simulink model "System2016"  (R2016b)
settings: Solver=ode45  StartTime=0.0  StopTime=3  RelTol=1e-3  EnableMultiTasking=on
libraries: powerlib x4, simulink x2, powerlib_meascontrol x1
settings Model: Creator=Administrator  LastModifiedBy=Administrator
settings DataIOCC: LimitDataPoints=on  SaveFormat=Array
settings OptimizationCC: LifeSpan=inf
settings DebuggingCC: SolverPrmCheckMsg=warning  SFUnexpectedBacktrackingDiag=warning  SFNoUnconditionalDefaultTransitionDiag=warning  SFExecutionAtInitializationDiag=none
settings HardwareCC: ProdBitPerPointer=32  ProdBitPerSizeT=32  ProdBitPerPtrDiffT=32  ProdLargestAtomicFloat=None  ProdIntDivRoundTo=Undefined  ProdEndianess=Unspecified  ProdWordSize=32  ProdHWDeviceType=32-bit Generic
settings ModelReferenceCC: PropagateSignalLabelsOutOfModel=off
settings GRTTargetCC: TargetLangStandard=C89/C90 (ANSI)  GeneratePreprocessorConditionals=Disable all
settings ConfigComp: CovMetricSettings=dw  CovHtmlReporting=on  CovSaveCumulativeToWorkspaceVar=on  CovSaveSingleToWorkspaceVar=on  CovExternalEMLEnable=off  CovSFcnEnable=off

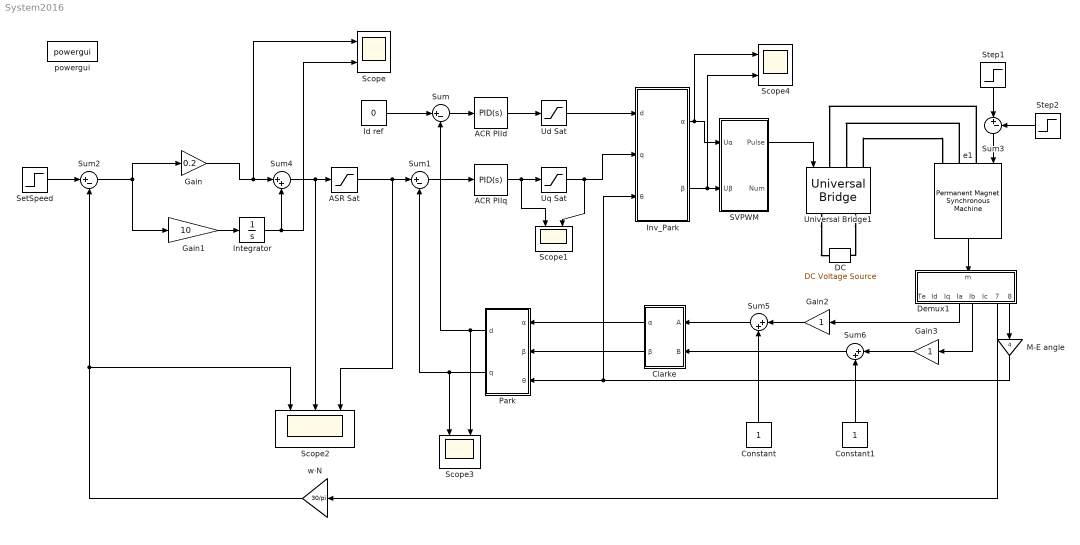
== system System2016 ==
  " e1" : powerlib/Machines/Permanent Magnet Synchronous Machine  NbPhases=3  FluxDistribution=Sinusoidal  RotorType=Round  MechanicalLoad=Torque Tm  PresetModel=No  ShowDetailedParameters=on  MeasurementBus=off  Resistance=1  Inductance=8.5e-3  dqInductances=[8.5e-3,8.5e-3]  La=0.01  MachineConstant=Flux linkage established by magnets (V.s)  Flux=0.1827  VoltageCst=132.5525  TorqueCst=1.0962  Flat=120  Mechanical=[0.006 0.0003035 4 0]  PolePairs=4  InitialConditions=[0,0, 0,0]  InitialConditions5ph=[0 0 0 0 0 0]  TsPowergui=0  TsBlock=-1  RefAngle=Aligned with phase A axis (original Park)
  ACR PIId : simulink/Continuous/PID Controller  Controller=PID  TimeDomain=Continuous-time  SampleTime=-1  IntegratorMethod=Forward Euler  FilterMethod=Forward Euler  Form=Parallel  UseFilter=on  ControllerParametersSource=internal  P=45  I=23  D=0  N=100  InitialConditionSource=internal  InitialConditionForIntegrator=0  InitialConditionForFilter=0  ExternalReset=none  LimitOutput=off  UpperSaturationLimit=inf  LowerSaturationLimit=-inf  LinearizeAsGain=on  AntiWindupMode=none  Kb=1  TrackingMode=off  Kt=1  PParamMin=[]  PParamMax=[]  IParamMin=[]  IParamMax=[]  DParamMin=[]  DParamMax=[]  NParamMin=[]  NParamMax=[]  KbParamMin=[]  KbParamMax=[]  KtParamMin=[]  KtParamMax=[]  POutMin=[]  POutMax=[]  IOutMin=[]  IOutMax=[]  DOutMin=[]  DOutMax=[]  NOutMin=[]  NOutMax=[]  KbOutMin=[]  KbOutMax=[]  KtOutMin=[]  KtOutMax=[]  IntegratorOutMin=[]  IntegratorOutMax=[]  FilterOutMin=[]  FilterOutMax=[]  SumOutMin=[]  SumOutMax=[]  SumI1OutMin=[]  SumI1OutMax=[]  SumI2OutMin=[]  SumI2OutMax=[]  SumI3OutMin=[]  SumI3OutMax=[]  SumDOutMin=[]  SumDOutMax=[]  SaturationOutMin=[]  SaturationOutMax=[]  IntegratorContinuousStateAttributes=''  IntegratorStateMustResolveToSignalObject=off  IntegratorRTWStateStorageClass=Auto  FilterContinuousStateAttributes=''  FilterStateMustResolveToSignalObject=off  FilterRTWStateStorageClass=Auto  DifferentiatorICPrevScaledInput=0  DifferentiatorOutMin=[]  DifferentiatorOutMax=[]
  ACR PIIq : simulink/Continuous/PID Controller  Controller=PID  TimeDomain=Continuous-time  SampleTime=-1  IntegratorMethod=Forward Euler  FilterMethod=Forward Euler  Form=Parallel  UseFilter=on  ControllerParametersSource=internal  P=32  I=23  D=0  N=100  InitialConditionSource=internal  InitialConditionForIntegrator=0  InitialConditionForFilter=0  ExternalReset=none  LimitOutput=off  UpperSaturationLimit=inf  LowerSaturationLimit=-inf  LinearizeAsGain=on  AntiWindupMode=none  Kb=1  TrackingMode=off  Kt=1  PParamMin=[]  PParamMax=[]  IParamMin=[]  IParamMax=[]  DParamMin=[]  DParamMax=[]  NParamMin=[]  NParamMax=[]  KbParamMin=[]  KbParamMax=[]  KtParamMin=[]  KtParamMax=[]  POutMin=[]  POutMax=[]  IOutMin=[]  IOutMax=[]  DOutMin=[]  DOutMax=[]  NOutMin=[]  NOutMax=[]  KbOutMin=[]  KbOutMax=[]  KtOutMin=[]  KtOutMax=[]  IntegratorOutMin=[]  IntegratorOutMax=[]  FilterOutMin=[]  FilterOutMax=[]  SumOutMin=[]  SumOutMax=[]  SumI1OutMin=[]  SumI1OutMax=[]  SumI2OutMin=[]  SumI2OutMax=[]  SumI3OutMin=[]  SumI3OutMax=[]  SumDOutMin=[]  SumDOutMax=[]  SaturationOutMin=[]  SaturationOutMax=[]  IntegratorContinuousStateAttributes=''  IntegratorStateMustResolveToSignalObject=off  IntegratorRTWStateStorageClass=Auto  FilterContinuousStateAttributes=''  FilterStateMustResolveToSignalObject=off  FilterRTWStateStorageClass=Auto  DifferentiatorICPrevScaledInput=0  DifferentiatorOutMin=[]  DifferentiatorOutMax=[]
  ASR Sat : Saturate  UpperLimit=2  LowerLimit=-2
  Clarke : Subsystem
  Constant : Constant
  Constant1 : Constant
  DC : powerlib/Electrical Sources/DC Voltage Source  Amplitude=50  Measurements=None
  Demux1 : Subsystem
  Gain : Gain  Gain=0.2
  Gain1 : Gain  Gain=10
  Gain2 : Gain
  Gain3 : Gain
  Id ref : Constant  Value=0
  Integrator : Integrator
  Inv_Park : Subsystem
  M-E angle : Gain  Gain=4
  Park : Subsystem
  "SVPWM " : Subsystem
  Scope{,1,3..4} (4 alike) : Scope  NumInputPorts=2
  Scope2 : Scope  NumInputPorts=3
  SetSpeed : Step  Time=0  Before=40  After=40  SampleTime=0
  Step1 : Step  Before=1  After=1.5  SampleTime=0
  Step2 : Step  Time=1.05  After=0.5  SampleTime=0
  Sum{,1..3} (4 alike) : Sum  Inputs=|+-
  Sum4 : Sum  Inputs=|++
  Sum5 : Sum  Inputs=|++
  Sum6 : Sum  Inputs=|++
  Ud Sat : Saturate  UpperLimit=38  LowerLimit=-38
  Universal Bridge1 : powerlib/Power Electronics/Universal Bridge  Arms=3  SnubberResistance=1e5  SnubberCapacitance=inf  Device=IGBT / Diodes  Ron=1e-3  Lon=0  ForwardVoltages="[  0  0  ]"  ForwardVoltage=0  GTOparameters=[ 10e-6 , 20e-6 ]  IGBTparameters=[ 1e-6 , 2e-6 ]  Measurements=None  Measurements_2=None  converterType=Rectifier
  Uq Sat : Saturate  UpperLimit=38  LowerLimit=-38
  powergui : powerlib/powergui  SimulationMode=Continuous  SolverType=Tustin  SampleTime=50e-6  frequency=60  SPID=off  DisableSnubberDevices=off  DisableRonSwitches=off  DisableVfSwitches=off  SwTol=0  DisplayEquations=off  Interpol=off  ExternalGateDelay=off  methode=off  Ts=0  FunctionMessages=off  echomessages=off  HookPort=off  EnableUseOfTLC=off  x0status=blocks  frequencyindice=0  Pbase=100e6  ErrMax=1e-4  Iterations=50  UnitsV=kV  UnitsW=MW  buscounter=0  RestoreLinks=warning  ResistiveCurrentMeasurement=off  Frange=[0:2:500]  Ylog=off  Xlog=on  ShowGrid=off  save=off  variable=ZData  structure=0  ZoomFFT=on  StartTime=0.0  cycles=1  DisplayStyle=1  fundamental=60  FreqAxis=off  MaxFrequency=1000  frequencyindicesteady=1  RmsSteady=1  display=off
  w·N : Gain  Gain=30/pi
  wires:
  "SVPWM "/1(Pulse) -> Universal Bridge1/1
  Inv_Park/1(α) -> Scope4/1, "SVPWM "/1(Uα)
  Inv_Park/2(β) -> Scope4/2, "SVPWM "/2(Uβ)
  Sum/1 -> ACR PIId/1
  Sum1/1 -> ACR PIIq/1
  Id ref/1 -> Sum/1
  SetSpeed/1 -> Sum2/1
  Demux1/8(thetam) -> M-E angle/1
  Demux1/7(wm) -> w·N/1
  " e1"/1 -> Demux1/1(m)
  M-E angle/1 -> Park/3(θ), Inv_Park/3(θ)
  Clarke/1(α) -> Park/1(α)
  Clarke/2(β) -> Park/2(β)
  w·N/1 -> Sum2/2, Scope2/1
  Ud Sat/1 -> Inv_Park/1(d)
  Uq Sat/1 -> Scope1/2, Inv_Park/2(q)
  ACR PIIq/1 -> Scope1/1, Uq Sat/1
  ACR PIId/1 -> Ud Sat/1
  Park/1(d) -> Scope3/2, Sum/2
  Park/2(q) -> Scope3/1, Sum1/2
  ASR Sat/1 -> Scope2/3, Sum1/1
  Step1/1 -> Sum3/1
  Sum3/1 -> " e1"/1
  Step2/1 -> Sum3/2
  Sum4/1 -> Scope2/2, ASR Sat/1
  Integrator/1 -> Scope/2, Sum4/2
  Gain1/1 -> Integrator/1
  Sum2/1 -> Gain/1, Gain1/1
  Gain/1 -> Scope/1, Sum4/1
  Sum5/1 -> Clarke/1(A)
  Sum6/1 -> Clarke/2(B)
  Demux1/5(Ib) -> Gain3/1
  Demux1/4(Ia) -> Gain2/1
  Gain2/1 -> Sum5/1
  Gain3/1 -> Sum6/1
  Constant/1 -> Sum5/2
  Constant1/1 -> Sum6/2
  connections:
  " e1"/LConn1 -- Universal Bridge1/LConn1
  " e1"/LConn2 -- Universal Bridge1/LConn2
  Universal Bridge1/LConn3 -- " e1"/LConn3
  Universal Bridge1/RConn1 -- DC/RConn1
  Universal Bridge1/RConn2 -- DC/LConn1

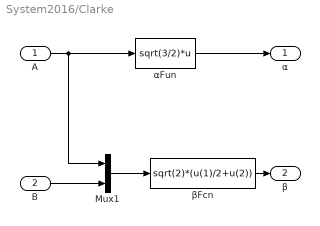
== system System2016/Clarke ==
  A : Inport
  B : Inport  Port=2
  Mux1 : Mux  Inputs=2
  αFun : Fcn  Expr=sqrt(3/2)*u
  βFcn : Fcn  Expr=sqrt(2)*(u(1)/2+u(2))
  α : Outport
  β : Outport  Port=2
  wires:
  A/1 -> Mux1/1, αFun/1
  αFun/1 -> α/1
  B/1 -> Mux1/2
  Mux1/1 -> βFcn/1
  βFcn/1 -> β/1

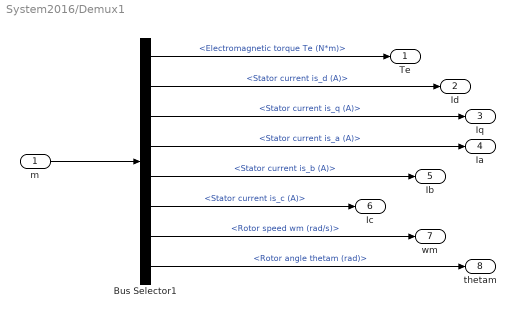
== system System2016/Demux1 ==
  m : Inport
  Bus Selector1 : BusSelector  OutputSignals=Electromagnetic torque Te (N*m),Stator current is_d (A),Stator current is_q (A),Stator current is_a (A),Stator current is_b (A),Stator current is_c (A),Rotor speed wm (rad/s),Rotor angle thetam (rad)
  Te : Outport
  Id : Outport  Port=2
  Iq : Outport  Port=3
  Ia : Outport  Port=4
  Ib : Outport  Port=5
  Ic : Outport  Port=6
  wm : Outport  Port=7
  thetam : Outport  Port=8
  wires:
  m/1 -> Bus Selector1/1
  Bus Selector1/4 -> Ia/1  "<Stator current is_a (A)>"
  Bus Selector1/5 -> Ib/1  "<Stator current is_b (A)>"
  Bus Selector1/6 -> Ic/1  "<Stator current is_c (A)>"
  Bus Selector1/7 -> wm/1  "<Rotor speed wm (rad/s)>"
  Bus Selector1/8 -> thetam/1  "<Rotor angle thetam (rad)>"
  Bus Selector1/1 -> Te/1  "<Electromagnetic torque Te (N*m)>"
  Bus Selector1/2 -> Id/1  "<Stator current is_d (A)>"
  Bus Selector1/3 -> Iq/1  "<Stator current is_q (A)>"

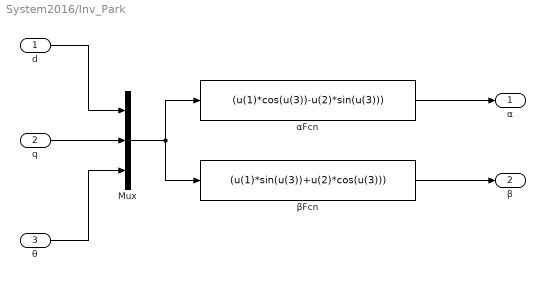
== system System2016/Inv_Park ==
  d : Inport
  q : Inport  Port=2
  θ : Inport  Port=3
  Mux : Mux  Inputs=3
  αFcn : Fcn  Expr=(u(1)*cos(u(3))-u(2)*sin(u(3)))
  βFcn : Fcn  Expr=(u(1)*sin(u(3))+u(2)*cos(u(3)))
  α : Outport
  β : Outport  Port=2
  wires:
  d/1 -> Mux/1
  q/1 -> Mux/2
  θ/1 -> Mux/3
  αFcn/1 -> α/1
  βFcn/1 -> β/1
  Mux/1 -> βFcn/1, αFcn/1

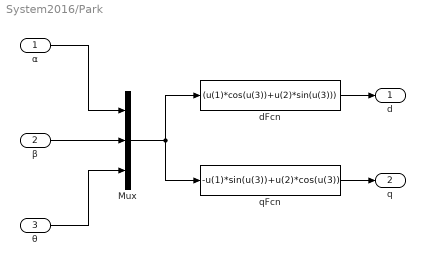
== system System2016/Park ==
  α : Inport
  β : Inport  Port=2
  θ : Inport  Port=3
  Mux : Mux  Inputs=3
  dFcn : Fcn  Expr=(u(1)*cos(u(3))+u(2)*sin(u(3)))
  qFcn : Fcn  Expr=-u(1)*sin(u(3))+u(2)*cos(u(3))
  d : Outport
  q : Outport  Port=2
  wires:
  α/1 -> Mux/1
  β/1 -> Mux/2
  θ/1 -> Mux/3
  dFcn/1 -> d/1
  qFcn/1 -> q/1
  Mux/1 -> qFcn/1, dFcn/1

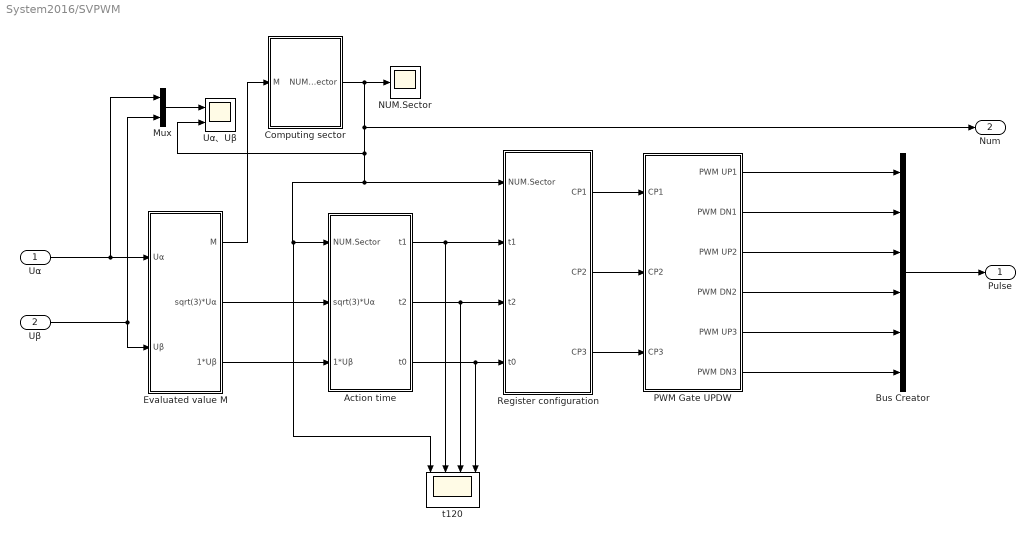
== system System2016/SVPWM  ==
  Uα : Inport
  Uβ : Inport  Port=2
  Action time : Subsystem
  Bus Creator : BusCreator  Inputs=6
  Computing sector : Subsystem
  Evaluated value M : Subsystem
  Mux : Mux  Inputs=2
  NUM.Sector : Scope
  PWM Gate UPDW : Subsystem
  Register configuration : Subsystem
  Uα、Uβ : Scope  NumInputPorts=2
  t120 : Scope  NumInputPorts=4
  Pulse : Outport
  Num : Outport  Port=2
  wires:
  Evaluated value M/1(M) -> Computing sector/1(M)
  Computing sector/1(NUM.Sector) -> NUM.Sector/1, Num/1, Uα、Uβ/2, t120/1, Action time/1(NUM.Sector), Register configuration/1(NUM.Sector)
  Evaluated value M/2(sqrt(3)*Uα) -> Action time/2(sqrt(3)*Uα)
  Evaluated value M/3(1*Uβ) -> Action time/3(1*Uβ)
  Action time/1(t1) -> t120/2, Register configuration/2(t1)
  Action time/2(t2) -> t120/3, Register configuration/3(t2)
  Action time/3(t0) -> t120/4, Register configuration/4(t0)
  Register configuration/1(CP1) -> PWM Gate UPDW/1(CP1)
  Register configuration/2(CP2) -> PWM Gate UPDW/2(CP2)
  Register configuration/3(CP3) -> PWM Gate UPDW/3(CP3)
  PWM Gate UPDW/1(PWM UP1) -> Bus Creator/1
  Uα/1 -> Mux/1, Evaluated value M/1(Uα)
  Uβ/1 -> Mux/2, Evaluated value M/2(Uβ)
  Mux/1 -> Uα、Uβ/1
  Bus Creator/1 -> Pulse/1
  PWM Gate UPDW/2(PWM DN1) -> Bus Creator/2
  PWM Gate UPDW/3(PWM UP2) -> Bus Creator/3
  PWM Gate UPDW/4(PWM DN2) -> Bus Creator/4
  PWM Gate UPDW/5(PWM UP3) -> Bus Creator/5
  PWM Gate UPDW/6(PWM DN3) -> Bus Creator/6

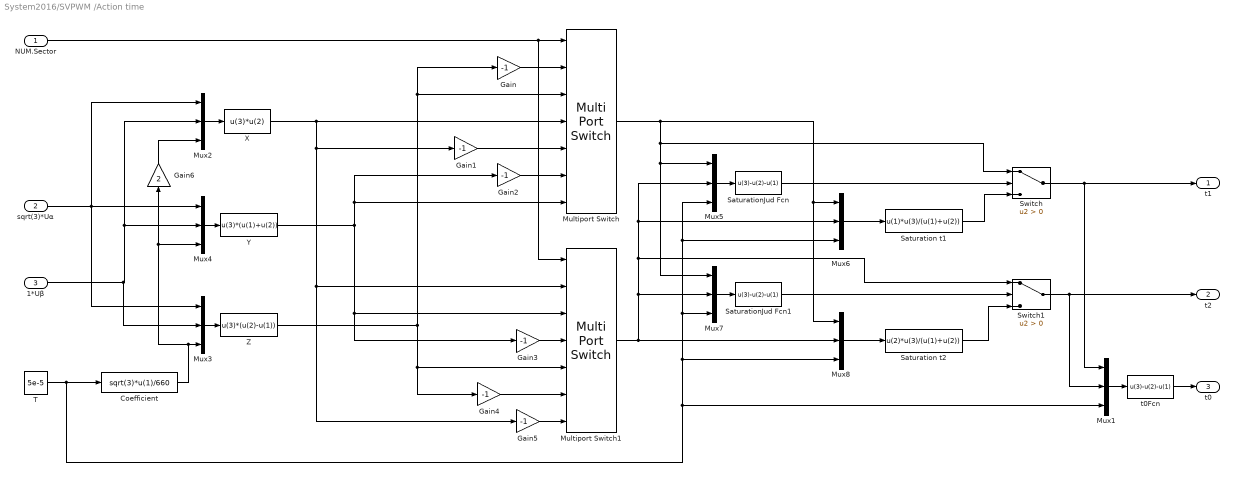
== system System2016/SVPWM /Action time ==
  NUM.Sector : Inport
  sqrt(3)*Uα : Inport  Port=2
  1*Uβ : Inport  Port=3
  Coefficient : Fcn  Expr=sqrt(3)*u(1)/660
  Gain{,1..5} (6 alike) : Gain  Gain=-1
  Gain6 : Gain  Gain=2
  Multiport Switch : MultiPortSwitch  Inputs=6
  Multiport Switch1 : MultiPortSwitch  Inputs=6
  Mux{1..8} (8 alike) : Mux  Inputs=3
  Saturation t1 : Fcn  Expr=u(1)*u(3)/(u(1)+u(2))
  Saturation t2 : Fcn  Expr=u(2)*u(3)/(u(1)+u(2))
  SaturationJud Fcn : Fcn  Expr=u(3)-u(2)-u(1)
  SaturationJud Fcn1 : Fcn  Expr=u(3)-u(2)-u(1)
  Switch : Switch  Criteria=u2 > Threshold
  Switch1 : Switch  Criteria=u2 > Threshold
  T : Constant  Value=5e-5
  X : Fcn  Expr=u(3)*u(2)
  Y : Fcn  Expr=u(3)*(u(1)+u(2))
  Z : Fcn  Expr=u(3)*(u(2)-u(1))
  t0Fcn : Fcn  Expr=u(3)-u(2)-u(1)
  t1 : Outport
  t2 : Outport  Port=2
  t0 : Outport  Port=3
  wires:
  NUM.Sector/1 -> Multiport Switch1/1, Multiport Switch/1
  T/1 -> Coefficient/1, Mux1/3, Mux8/3, Mux7/3, Mux5/3, Mux6/3
  Mux1/1 -> t0Fcn/1
  t0Fcn/1 -> t0/1
  sqrt(3)*Uα/1 -> Mux3/1, Mux4/1, Mux2/1
  1*Uβ/1 -> Mux3/2, Mux4/2, Mux2/2
  Coefficient/1 -> Mux4/3, Gain6/1, Mux3/3
  Mux2/1 -> X/1
  Mux4/1 -> Y/1
  Mux3/1 -> Z/1
  Gain/1 -> Multiport Switch/2
  Gain1/1 -> Multiport Switch/5
  Gain2/1 -> Multiport Switch/6
  Gain3/1 -> Multiport Switch1/4
  Gain4/1 -> Multiport Switch1/6
  Gain5/1 -> Multiport Switch1/7
  Z/1 -> Gain/1, Multiport Switch/3, Multiport Switch1/5, Gain4/1
  X/1 -> Gain1/1, Multiport Switch1/2, Gain5/1, Multiport Switch/4
  Y/1 -> Multiport Switch/7, Gain2/1, Gain3/1, Multiport Switch1/3
  Multiport Switch/1 -> Mux8/1, Mux6/1, Switch/1, Mux7/1, Mux5/1
  Multiport Switch1/1 -> Mux7/2, Switch1/1, Mux6/2, Mux5/2, Mux8/2
  Mux5/1 -> SaturationJud Fcn/1
  SaturationJud Fcn/1 -> Switch/2
  Switch/1 -> Mux1/1, t1/1
  Saturation t1/1 -> Switch/3
  Mux6/1 -> Saturation t1/1
  Mux7/1 -> SaturationJud Fcn1/1
  Switch1/1 -> Mux1/2, t2/1
  Mux8/1 -> Saturation t2/1
  SaturationJud Fcn1/1 -> Switch1/2
  Saturation t2/1 -> Switch1/3
  Gain6/1 -> Mux2/3

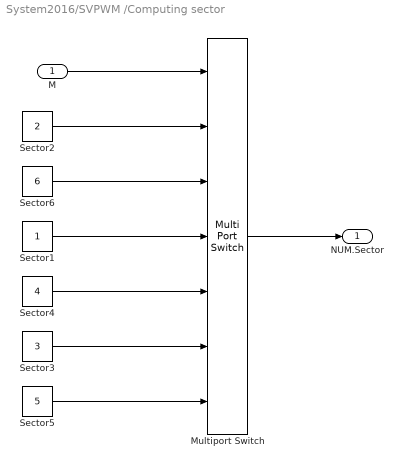
== system System2016/SVPWM /Computing sector ==
  M : Inport
  Multiport Switch : MultiPortSwitch  Inputs=6
  Sector1 : Constant
  Sector2 : Constant  Value=2
  Sector3 : Constant  Value=3
  Sector4 : Constant  Value=4
  Sector5 : Constant  Value=5
  Sector6 : Constant  Value=6
  NUM.Sector : Outport
  wires:
  M/1 -> Multiport Switch/1
  Sector2/1 -> Multiport Switch/2
  Sector6/1 -> Multiport Switch/3
  Sector1/1 -> Multiport Switch/4
  Sector4/1 -> Multiport Switch/5
  Sector3/1 -> Multiport Switch/6
  Sector5/1 -> Multiport Switch/7
  Multiport Switch/1 -> NUM.Sector/1

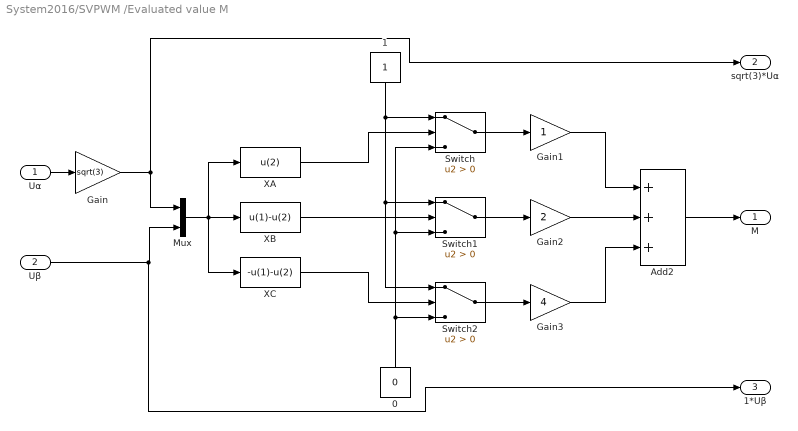
== system System2016/SVPWM /Evaluated value M ==
  Uα : Inport
  Uβ : Inport  Port=2
  0 : Constant  Value=0
  1 : Constant
  Add2 : Sum  Inputs=+++
  Gain : Gain  Gain=sqrt(3)
  Gain1 : Gain
  Gain2 : Gain  Gain=2
  Gain3 : Gain  Gain=4
  Mux : Mux  Inputs=2
  Switch : Switch  Criteria=u2 > Threshold
  Switch1 : Switch  Criteria=u2 > Threshold
  Switch2 : Switch  Criteria=u2 > Threshold
  XA : Fcn  Expr=u(2)
  XB : Fcn  Expr=u(1)-u(2)
  XC : Fcn  Expr=-u(1)-u(2)
  M : Outport
  sqrt(3)*Uα : Outport  Port=2
  1*Uβ : Outport  Port=3
  wires:
  Uβ/1 -> 1*Uβ/1, Mux/2
  Mux/1 -> XA/1, XB/1, XC/1
  XB/1 -> Switch1/2
  XA/1 -> Switch/2
  XC/1 -> Switch2/2
  0/1 -> Switch2/3, Switch1/3, Switch/3
  1/1 -> Switch/1, Switch1/1, Switch2/1
  Switch/1 -> Gain1/1
  Switch1/1 -> Gain2/1
  Switch2/1 -> Gain3/1
  Gain1/1 -> Add2/1
  Gain2/1 -> Add2/2
  Gain3/1 -> Add2/3
  Add2/1 -> M/1
  Uα/1 -> Gain/1
  Gain/1 -> Mux/1, sqrt(3)*Uα/1

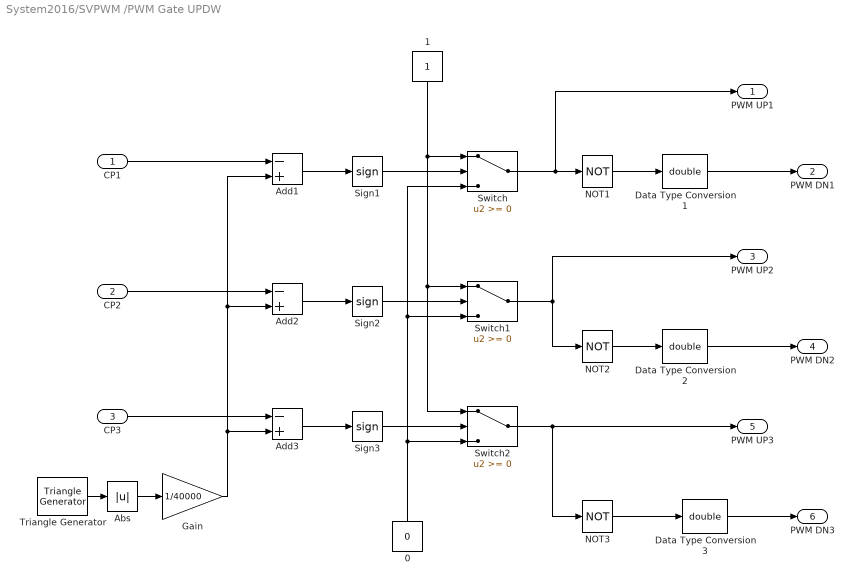
== system System2016/SVPWM /PWM Gate UPDW ==
  CP1 : Inport
  CP2 : Inport  Port=2
  CP3 : Inport  Port=3
  0 : Constant  Value=0
  1 : Constant
  Abs : Abs
  Add1 : Sum  Inputs=-+
  Add2 : Sum  Inputs=-+
  Add3 : Sum  Inputs=-+
  Data Type Conversion1 : DataTypeConversion  OutDataTypeStr=double
  Data Type Conversion2 : DataTypeConversion  OutDataTypeStr=double
  Data Type Conversion3 : DataTypeConversion  OutDataTypeStr=double
  Gain : Gain  Gain=1/40000
  NOT1 : Logic  Operator=NOT  AllPortsSameDT=off  OutDataTypeStr=boolean
  NOT2 : Logic  Operator=NOT  AllPortsSameDT=off  OutDataTypeStr=boolean
  NOT3 : Logic  Operator=NOT  AllPortsSameDT=off  OutDataTypeStr=boolean
  Sign1 : Signum
  Sign2 : Signum
  Sign3 : Signum
  Switch : Switch
  Switch1 : Switch
  Switch2 : Switch
  Triangle Generator : powerlib_meascontrol/Pulse & Signal Generators/Triangle Generator  Freq=1e4  Phase=90  Ts=0
  PWM UP1 : Outport
  PWM DN1 : Outport  Port=2
  PWM UP2 : Outport  Port=3
  PWM DN2 : Outport  Port=4
  PWM UP3 : Outport  Port=5
  PWM DN3 : Outport  Port=6
  wires:
  1/1 -> Switch2/1, Switch1/1, Switch/1
  0/1 -> Switch2/3, Switch1/3, Switch/3
  Switch/1 -> PWM UP1/1, NOT1/1
  Switch1/1 -> NOT2/1, PWM UP2/1
  Switch2/1 -> PWM UP3/1, NOT3/1
  Sign1/1 -> Switch/2
  Sign2/1 -> Switch1/2
  Sign3/1 -> Switch2/2
  Add3/1 -> Sign3/1
  Add2/1 -> Sign2/1
  Add1/1 -> Sign1/1
  CP1/1 -> Add1/1
  CP2/1 -> Add2/1
  CP3/1 -> Add3/1
  Gain/1 -> Add3/2, Add2/2, Add1/2
  Triangle Generator/1 -> Abs/1
  Abs/1 -> Gain/1
  NOT1/1 -> Data Type Conversion1/1
  NOT2/1 -> Data Type Conversion2/1
  Data Type Conversion2/1 -> PWM DN2/1
  NOT3/1 -> Data Type Conversion3/1
  Data Type Conversion3/1 -> PWM DN3/1
  Data Type Conversion1/1 -> PWM DN1/1

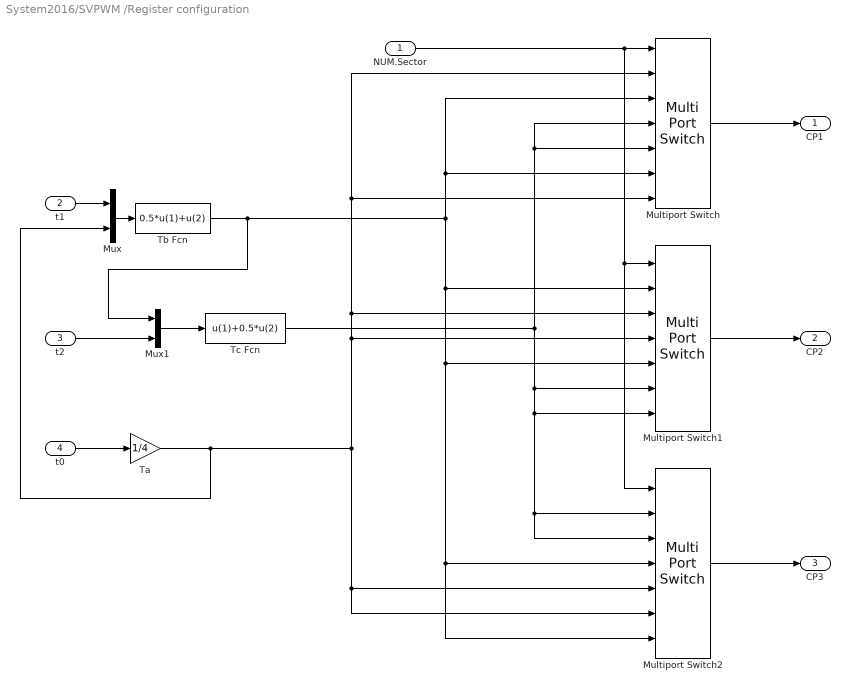
== system System2016/SVPWM /Register configuration ==
  NUM.Sector : Inport
  t1 : Inport  Port=2
  t2 : Inport  Port=3
  t0 : Inport  Port=4
  Multiport Switch : MultiPortSwitch  Inputs=6
  Multiport Switch1 : MultiPortSwitch  Inputs=6
  Multiport Switch2 : MultiPortSwitch  Inputs=6
  Mux : Mux  Inputs=2
  Mux1 : Mux  Inputs=2
  Ta : Gain  Gain=1/4
  Tb Fcn : Fcn  Expr=0.5*u(1)+u(2)
  Tc Fcn : Fcn  Expr=u(1)+0.5*u(2)
  CP1 : Outport
  CP2 : Outport  Port=2
  CP3 : Outport  Port=3
  wires:
  t0/1 -> Ta/1
  NUM.Sector/1 -> Multiport Switch2/1, Multiport Switch1/1, Multiport Switch/1
  Multiport Switch/1 -> CP1/1
  Multiport Switch1/1 -> CP2/1
  Multiport Switch2/1 -> CP3/1
  t1/1 -> Mux/1
  Ta/1 -> Mux/2, Multiport Switch2/6, Multiport Switch2/5, Multiport Switch1/4, Multiport Switch1/3, Multiport Switch/7, Multiport Switch/2
  Mux/1 -> Tb Fcn/1
  t2/1 -> Mux1/2
  Mux1/1 -> Tc Fcn/1
  Tc Fcn/1 -> Multiport Switch/5, Multiport Switch/4, Multiport Switch2/3, Multiport Switch2/2, Multiport Switch1/7, Multiport Switch1/6
  Tb Fcn/1 -> Multiport Switch/6, Multiport Switch/3, Multiport Switch1/5, Multiport Switch2/7, Multiport Switch2/4, Multiport Switch1/2, Mux1/1
